simulink model "ArrayAvg"  (R2021a)
settings: Solver=FixedStepDiscrete  StartTime=0.0  StopTime=10.0  RelTol=1e-3  EnableMultiTasking=on
settings Model: Creator=Momen El Sayed  LastModifiedBy=Momen El Sayed
settings DataIOCC: ReturnWorkspaceOutputs=off
settings OptimizationCC: DefaultParameterBehavior=Inlined  InlineInvariantSignals=on  EnableMemcpy=off  LifeSpan=1  EfficientTunableParamExpr=on
settings DebuggingCC: UnderspecifiedInitializationDetection=Classic  MergeDetectMultiDrivingBlocksExec=none  SFMachineParentedDataDiag=warning  ArithmeticOperatorsInVariantConditions=warning
settings ModelReferenceCC: PropagateSignalLabelsOutOfModel=off
settings SFSimCC: MATLABDynamicMemAlloc=off  CustomCodeUndefinedFunction=UseInterfaceOnly
settings RTWCC: SystemTargetFile=ert.tlc  GenCodeOnly=on  TemplateMakefile=ert_default_tmf  GenerateReport=on  IncludeHyperlinkInReport=on  LaunchReport=on  GenerateTraceInfo=on  GenerateTraceReport=on  GenerateTraceReportSl=on  GenerateTraceReportSf=on  GenerateTraceReportEml=on
settings CodeAppCC: ForceParamTrailComments=on  IgnoreCustomStorageClasses=off  OperatorAnnotations=on  SimulinkDataObjDesc=on  SFDataObjDesc=on  MATLABFcnDesc=on  InsertBlockDesc=on  StateflowObjectComments=on  MATLABSourceComments=on
settings ERTTargetCC: MultiwordLength=2048  GenerateSampleERTMain=on  InlinedParameterPlacement=NonHierarchical  ERTCustomFileTemplate=example_file_process.tlc

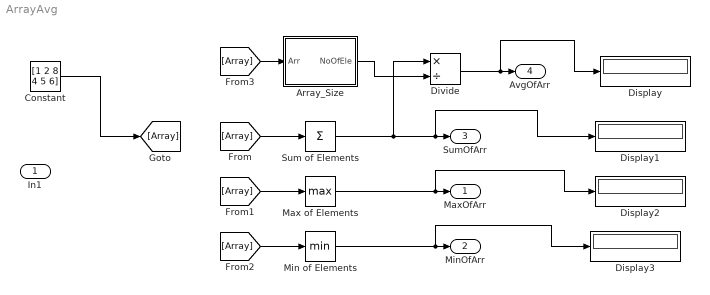
== system ArrayAvg ==
  In1 : Inport  PortDimensions=10
  Array_Size : MATLAB Function  TreatAsAtomicUnit=on
  Constant : Constant  Value=[1 2 8 4 5 6]
  Display{,1..3} (4 alike) : Display
  Divide : Product  Inputs=*/
  Max of Elements : MinMax  Function=max
  Min of Elements : MinMax
  Sum of Elements : Sum  Inputs=+
  MaxOfArr : Outport
  MinOfArr : Outport  Port=2
  SumOfArr : Outport  Port=3
  AvgOfArr : Outport  Port=4
  wires:
  Constant/1 -> [Array]
  [Array] -> Sum of Elements/1
  [Array] -> Max of Elements/1
  [Array] -> Min of Elements/1
  [Array] -> Array_Size/1(Arr)
  Sum of Elements/1 -> Display1/1, SumOfArr/1, Divide/1
  Array_Size/1(NoOfEle) -> Divide/2
  Divide/1 -> Display/1, AvgOfArr/1
  Max of Elements/1 -> Display2/1, MaxOfArr/1
  Min of Elements/1 -> Display3/1, MinOfArr/1

== matlab function ArrayAvg/Array_Size ==
  data: Arr input; NoOfEle output
function NoOfEle = fcn(Arr)
    NoOfEle = length(Arr);
